simulink model "test_sf_tm_turb"  (R2012b)
settings: Solver=FixedStepDiscrete  StartTime=0.0  StopTime=1  FixedStep=1/1200  RelTol=1e-3
settings Model: Creator=HSidaoui  LastModifiedBy=hsidaoui

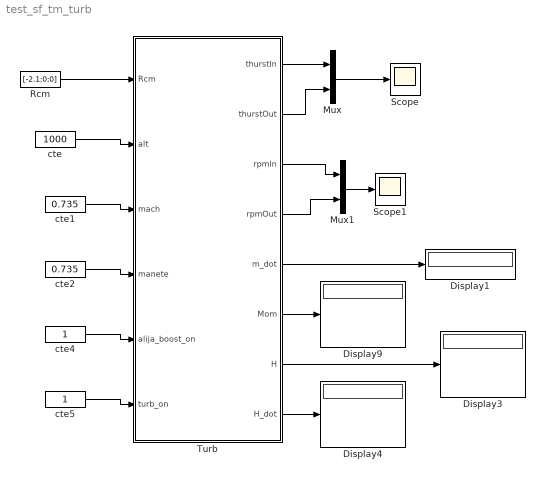
== system test_sf_tm_turb ==
  Display{1,3..4,9} (4 alike) : Display
  Mux : Mux  Inputs=2
  Mux1 : Mux  Inputs=2
  Rcm : Constant  Value=[-2.1;0;0]
  Scope : Scope
  Scope1 : Scope
  Turb : Subsystem  TreatAsAtomicUnit=on
  cte : Constant  Value=1000
  cte1 : Constant  Value=0.735
  cte2 : Constant  Value=0.735
  cte4 : Constant
  cte5 : Constant
  wires:
  cte/1 -> Turb/2(alt)
  Turb/1(thurstIn) -> Mux/1
  Turb/5(m_dot) -> Display1/1
  Turb/3(rpmIn) -> Mux1/1
  cte1/1 -> Turb/3(mach)
  Turb/6(Mom) -> Display9/1
  Rcm/1 -> Turb/1(Rcm)
  cte2/1 -> Turb/4(manete)
  cte5/1 -> Turb/6(turb_on)
  cte4/1 -> Turb/5(alija_boost_on)
  Turb/7(H) -> Display3/1
  Turb/8(H_dot) -> Display4/1
  Turb/2(thurstOut) -> Mux/2
  Mux/1 -> Scope/1
  Turb/4(rpmOut) -> Mux1/2
  Mux1/1 -> Scope1/1

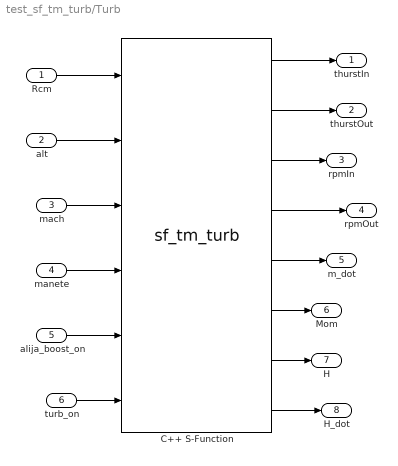
== system test_sf_tm_turb/Turb ==
  Rcm : Inport
  alt : Inport  Port=2
  mach : Inport  Port=3
  manete : Inport  Port=4
  alija_boost_on : Inport  Port=5
  turb_on : Inport  Port=6
  C++ S-Function : S-Function  FunctionName=sf_tm_turb  EnableBusSupport=off
  thurstIn : Outport
  thurstOut : Outport  Port=2
  rpmIn : Outport  Port=3
  rpmOut : Outport  Port=4
  m_dot : Outport  Port=5
  Mom : Outport  Port=6
  H : Outport  Port=7
  H_dot : Outport  Port=8
  wires:
  C++ S-Function/1 -> thurstIn/1
  Rcm/1 -> C++ S-Function/1
  alt/1 -> C++ S-Function/2
  mach/1 -> C++ S-Function/3
  manete/1 -> C++ S-Function/4
  alija_boost_on/1 -> C++ S-Function/5
  turb_on/1 -> C++ S-Function/6
  C++ S-Function/2 -> thurstOut/1
  C++ S-Function/3 -> rpmIn/1
  C++ S-Function/4 -> rpmOut/1
  C++ S-Function/8 -> H_dot/1
  C++ S-Function/7 -> H/1
  C++ S-Function/6 -> Mom/1
  C++ S-Function/5 -> m_dot/1
